simulink model "model_am_scalar"  (R2025a)
settings: Solver=FixedStepAuto  StartTime=0.0  StopTime=6  FixedStep=0.0001  RelTol=1e-3
values from neighbouring files (symbols this model uses):
  f = 50    [parametres_AM.m]
  J = 0.00096 * 5    (= 0.0048)    [parametres_AM.m]
  L1 = Lh + L1sig    (= 0.579)    [parametres_AM.m]
  L2 = L1    (= 0.579)    [parametres_AM.m]
  Lh = 0.56    [parametres_AM.m]
  M = 3.7    [parametres_AM.m]
  p = 2    [parametres_AM.m]
  R1 = 7.03    [parametres_AM.m]
  R2 = 3.44    [parametres_AM.m]
  sig = 1 - (Lh^2 / (L1 * L2))    (= 0.0645535599763)    [parametres_AM.m]
  U = 380    [parametres_AM.m]
  w = 2 * pi / 60 * n    (= 297.40410454)    [parametres_AM.m]
libraries: simulink x1
settings Model: Creator=Kajo  LastModifiedBy=emaka
settings SolverCC: AlgebraicLoopSolver=TrustRegion
settings DataIOCC: SaveOutput=off  SignalLogging=off  DSMLogging=off  SaveTime=off  ReturnWorkspaceOutputs=off
settings DebuggingCC: UnconnectedInputMsg=warning  UnconnectedOutputMsg=warning  UnconnectedLineMsg=warning
settings ModelReferenceCC: EnableRefExpFcnMdlSchedulingChecks=on
settings RTWCC: GPUComputeCapability=3.5

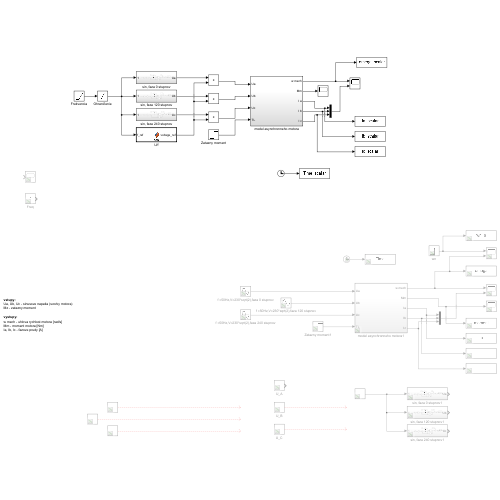
[thumbnail: Simulink's stored preview of the top-level diagram]
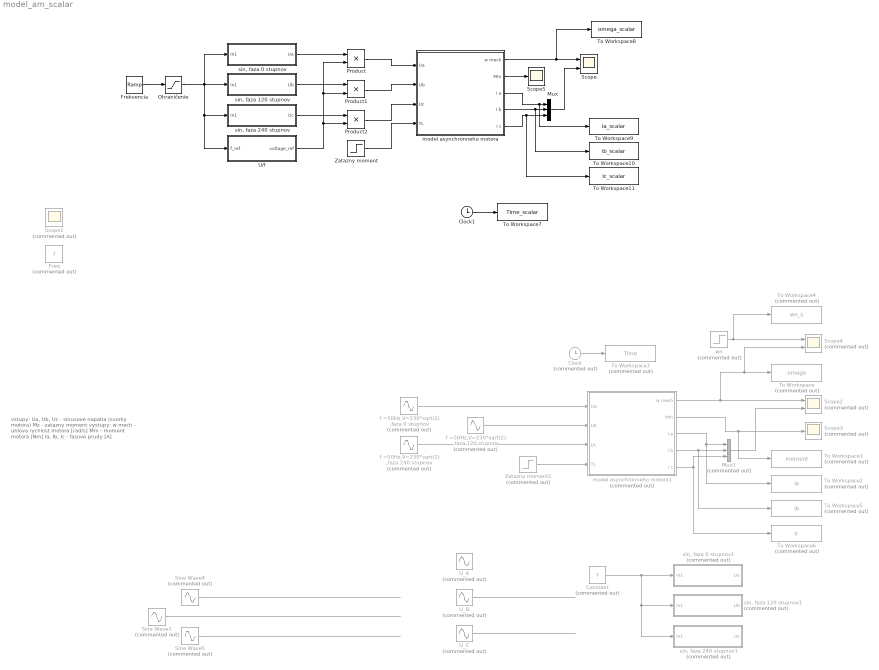
== system model_am_scalar ==
  note: vstupy:
      | Ua, Ub, Uc - sinusove napatia (svorky motora)
      | Mz - zatazny moment
      |
      | vystupy:
      | w mech - uhlova rychlost motora [rad/s]
      | Mm - moment motora [Nm]
      | Ia, Ib, Ic - fazove prudy [A]
  Clock : Clock  Commented=on
  Clock1 : Clock
  Constant : Constant  Commented=on  Value=f
  Frekvencia : simulink/Sources/Ramp  slope=16.67  start=0  InitialOutput=0
  Freq : Constant  Commented=on  Value=f  SampleTime=-1
  Mux : Mux  Inputs=3
  Mux1 : Mux  Commented=on  Inputs=3
  Ohraničenie : Saturate  UpperLimit=50  LowerLimit=0
  Product : Product
  Product1 : Product
  Product2 : Product
  Scope : Scope  NumInputPorts=2
      settings: ActiveDisplayYMinimum=-39.249692193358051  ActiveDisplayYMaximum=353.24722973603127
  Scope1 : Scope  Commented=on
      settings: ActiveDisplayYMinimum=-474.99354  ActiveDisplayYMaximum=474.99354
  Scope2 : Scope  Commented=on  NumInputPorts=2
      settings: ActiveDisplayYMinimum=-42.752099667675139  ActiveDisplayYMaximum=384.76889700905195  DataLoggingVariableName=ScopeData2
  Scope3 : Scope  Commented=on
      settings: ActiveDisplayYMinimum=-5.36519948546464  ActiveDisplayYMaximum=9.1078949851070767  DataLoggingVariableName=ScopeData3
  Scope4 : Scope  Commented=on  NumInputPorts=2
      settings: ActiveDisplayYMinimum=-1  ActiveDisplayYMaximum=1  DataLoggingVariableName=ScopeData4
  Scope5 : Scope
      settings: ActiveDisplayYMinimum=-0.94302291476539146  ActiveDisplayYMaximum=6.8461974059392778  DataLoggingVariableName=ScopeData6
  Sine Wave3 : Sin  Commented=on  Amplitude=U  Frequency=2*pi*50  SampleTime=0
  Sine Wave4 : Sin  Commented=on  Amplitude=U  Frequency=2*pi*50  Phase=(2*pi)/3  SampleTime=0
  Sine Wave5 : Sin  Commented=on  Amplitude=U  Frequency=2*pi*50  Phase=-(2*pi)/3  SampleTime=0
  To Workspace : ToWorkspace  Commented=on  VariableName=omega  SampleTime=-1
  To Workspace1 : ToWorkspace  Commented=on  VariableName=moment  SampleTime=-1
  To Workspace10 : ToWorkspace  VariableName=ib_scalar  SampleTime=-1
  To Workspace11 : ToWorkspace  VariableName=ic_scalar  SampleTime=-1
  To Workspace2 : ToWorkspace  Commented=on  VariableName=ia  SampleTime=-1
  To Workspace3 : ToWorkspace  Commented=on  VariableName=Time  SampleTime=-1
      settings: Save2DSignal=2-D array (concatenate along first dimension)
  To Workspace4 : ToWorkspace  Commented=on  VariableName=wn_s  SampleTime=-1
      settings: Save2DSignal=2-D array (concatenate along first dimension)
  To Workspace5 : ToWorkspace  Commented=on  VariableName=ib  SampleTime=-1
  To Workspace6 : ToWorkspace  Commented=on  VariableName=ic  SampleTime=-1
  To Workspace7 : ToWorkspace  VariableName=Time_scalar  SampleTime=-1
      settings: Save2DSignal=2-D array (concatenate along first dimension)
  To Workspace8 : ToWorkspace  VariableName=omega_scalar  SampleTime=-1
  To Workspace9 : ToWorkspace  VariableName=ia_scalar  SampleTime=-1
  U/f : MATLAB Function  TreatAsAtomicUnit=on
  U_A : Sin  Commented=on  Amplitude=U  Frequency=2*pi*f  SampleTime=0
  U_B : Sin  Commented=on  Amplitude=U  Frequency=2*pi*f  Phase=(2*pi)/3  SampleTime=0
  U_C : Sin  Commented=on  Amplitude=U  Frequency=2*pi*f  Phase=-(2*pi)/3  SampleTime=0
  Zatazny moment : Step  Time=4  After=M  SampleTime=0
  Zatazny moment1 : Step  Commented=on  After=M  SampleTime=0
  f =50Hz,V=230*sqrt(2),faza 0 stupnov : Sin  Commented=on  Amplitude=230*sqrt(2)  Frequency=2*pi*f  SampleTime=0
  f =50Hz,V=230*sqrt(2),faza 120 stupnov : Sin  Commented=on  Amplitude=230*sqrt(2)  Frequency=2*pi*f  Phase=-2*pi/3  SampleTime=0
  f =50Hz,V=230*sqrt(2),faza 240 stupnov : Sin  Commented=on  Amplitude=230*sqrt(2)  Frequency=2*pi*f  Phase=-4*pi/3  SampleTime=0
  model asynchronneho motora : Subsystem
  model asynchronneho motora1 : Subsystem  Commented=on
  "sin, faza 0 stupnov" : Subsystem
  "sin, faza 0 stupnov1" : Subsystem  Commented=on
  "sin, faza 120 stupnov" : Subsystem
  "sin, faza 120 stupnov1" : Subsystem  Commented=on
  "sin, faza 240 stupnov" : Subsystem
  "sin, faza 240 stupnov1" : Subsystem  Commented=on
  wn : Step  Commented=on  Time=0.01  After=w  SampleTime=0
  wires:
  Zatazny moment/1 -> model asynchronneho motora/4(TL)
  model asynchronneho motora/3(I a) -> To Workspace9/1, Mux/1
  model asynchronneho motora/4(I b) -> To Workspace10/1, Mux/2
  model asynchronneho motora/5(I c) -> To Workspace11/1, Mux/3
  Mux/1 -> Scope/2
  Product/1 -> model asynchronneho motora/1(Ua)
  Product1/1 -> model asynchronneho motora/2(Ub)
  Product2/1 -> model asynchronneho motora/3(Uc)
  "sin, faza 0 stupnov"/1(Ua) -> Product/1
  "sin, faza 120 stupnov"/1(Ub) -> Product1/1
  "sin, faza 240 stupnov"/1(Uc) -> Product2/1
  Ohraničenie/1 -> "sin, faza 0 stupnov"/1(In1), U/f/1(f_ref), "sin, faza 240 stupnov"/1(In1), "sin, faza 120 stupnov"/1(In1)
  Frekvencia/1 -> Ohraničenie/1
  U/f/1(voltage_ref) -> Product/2, Product1/2, Product2/2
  model asynchronneho motora1/4(I b) -> To Workspace5/1, Mux1/2
  model asynchronneho motora1/3(I a) -> Mux1/1, To Workspace2/1
  model asynchronneho motora1/5(I c) -> To Workspace6/1, Mux1/3
  Zatazny moment1/1 -> model asynchronneho motora1/4(TL)
  model asynchronneho motora1/1(w mech) -> Scope4/2, To Workspace/1, Scope2/1
  Mux1/1 -> Scope2/2
  U_C/1 -> ?
  U_B/1 -> ?
  Constant/1 -> "sin, faza 240 stupnov1"/1(In1), "sin, faza 120 stupnov1"/1(In1), "sin, faza 0 stupnov1"/1(In1)
  model asynchronneho motora1/2(Mm) -> To Workspace1/1, Scope3/1
  Sine Wave4/1 -> ?
  Sine Wave5/1 -> ?
  Sine Wave3/1 -> ?
  f =50Hz,V=230*sqrt(2),faza 0 stupnov/1 -> model asynchronneho motora1/1(Ua)
  f =50Hz,V=230*sqrt(2),faza 120 stupnov/1 -> model asynchronneho motora1/2(Ub)
  f =50Hz,V=230*sqrt(2),faza 240 stupnov/1 -> model asynchronneho motora1/3(Uc)
  wn/1 -> To Workspace4/1, Scope4/1
  Clock/1 -> To Workspace3/1
  model asynchronneho motora/2(Mm) -> Scope5/1
  Clock1/1 -> To Workspace7/1
  model asynchronneho motora/1(w mech) -> To Workspace8/1, Scope/1

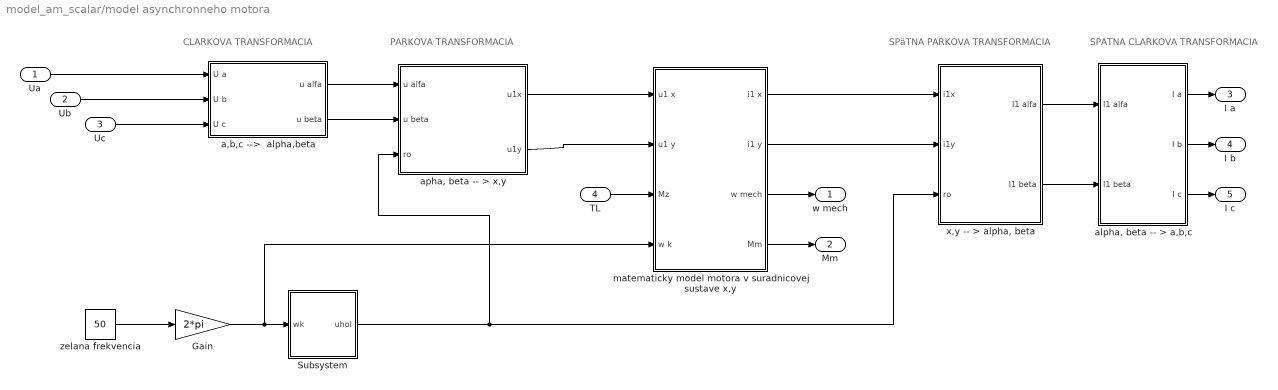
== system model_am_scalar/model asynchronneho motora ==
  note: PARKOVA TRANSFORMACIA
  note: SPATNA CLARKOVA TRANSFORMACIA
  note: SPäTNA PARKOVA TRANSFORMACIA
  note: CLARKOVA TRANSFORMACIA
  Ua : Inport
  Ub : Inport  Port=2
  Uc : Inport  Port=3
  TL : Inport  Port=4
  Gain : Gain  Gain=2*pi
  Subsystem : Subsystem
  "a,b,c -->  alpha,beta " : Subsystem
  "alpha, beta -- > a,b,c" : Subsystem
  "apha, beta -- > x,y" : Subsystem
  matematicky model motora v suradnicovej sustave x,y : Subsystem
  "x,y -- > alpha, beta" : Subsystem
  zelana frekvencia : Constant  Value=50
  w mech : Outport
  Mm : Outport  Port=2
  I a : Outport  Port=3
  I b : Outport  Port=4
  I c : Outport  Port=5
  wires:
  "a,b,c -->  alpha,beta "/1(u alfa) -> "apha, beta -- > x,y"/1(u alfa)
  "a,b,c -->  alpha,beta "/2(u beta) -> "apha, beta -- > x,y"/2(u beta)
  "apha, beta -- > x,y"/1(u1x) -> matematicky model motora v suradnicovej sustave x,y/1(u1 x)
  "apha, beta -- > x,y"/2(u1y) -> matematicky model motora v suradnicovej sustave x,y/2(u1 y)
  "x,y -- > alpha, beta"/1(I1 alfa) -> "alpha, beta -- > a,b,c"/1(I1 alfa)
  "x,y -- > alpha, beta"/2(I1 beta) -> "alpha, beta -- > a,b,c"/2(I1 beta)
  "alpha, beta -- > a,b,c"/1(I a) -> I a/1
  "alpha, beta -- > a,b,c"/2(I b) -> I b/1
  "alpha, beta -- > a,b,c"/3(I c) -> I c/1
  Ua/1 -> "a,b,c -->  alpha,beta "/1(U a)
  Ub/1 -> "a,b,c -->  alpha,beta "/2(U b)
  Uc/1 -> "a,b,c -->  alpha,beta "/3(U c)
  TL/1 -> matematicky model motora v suradnicovej sustave x,y/3(Mz)
  matematicky model motora v suradnicovej sustave x,y/2(i1 y) -> "x,y -- > alpha, beta"/2(i1y)
  matematicky model motora v suradnicovej sustave x,y/3(w mech) -> w mech/1
  matematicky model motora v suradnicovej sustave x,y/4(Mm) -> Mm/1
  matematicky model motora v suradnicovej sustave x,y/1(i1 x) -> "x,y -- > alpha, beta"/1(i1x)
  zelana frekvencia/1 -> Gain/1
  Gain/1 -> matematicky model motora v suradnicovej sustave x,y/4(w k), Subsystem/1(wk)
  Subsystem/1(uhol) -> "apha, beta -- > x,y"/3(ro), "x,y -- > alpha, beta"/3("ro ")

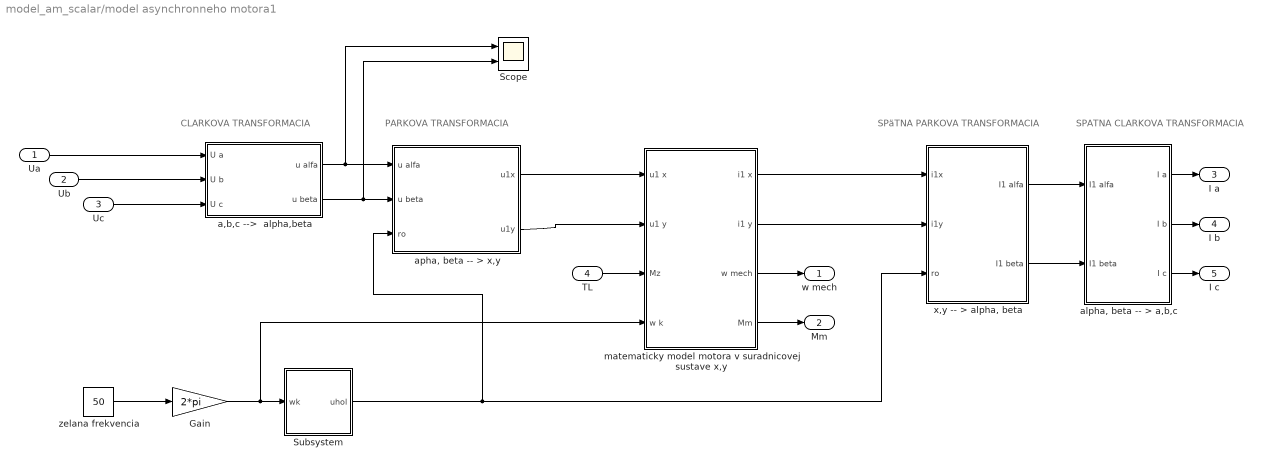
== system model_am_scalar/model asynchronneho motora1 ==
  note: PARKOVA TRANSFORMACIA
  note: SPATNA CLARKOVA TRANSFORMACIA
  note: SPäTNA PARKOVA TRANSFORMACIA
  note: CLARKOVA TRANSFORMACIA
  Ua : Inport
  Ub : Inport  Port=2
  Uc : Inport  Port=3
  TL : Inport  Port=4
  Gain : Gain  Gain=2*pi
  Scope : Scope  NumInputPorts=2
      settings: ActiveDisplayYMinimum=-412.2715694519627  ActiveDisplayYMaximum=371.70919052872546  DataLoggingVariableName=ScopeData5
  Subsystem : Subsystem
  "a,b,c -->  alpha,beta " : Subsystem
  "alpha, beta -- > a,b,c" : Subsystem
  "apha, beta -- > x,y" : Subsystem
  matematicky model motora v suradnicovej sustave x,y : Subsystem
  "x,y -- > alpha, beta" : Subsystem
  zelana frekvencia : Constant  Value=50
  w mech : Outport
  Mm : Outport  Port=2
  I a : Outport  Port=3
  I b : Outport  Port=4
  I c : Outport  Port=5
  wires:
  "a,b,c -->  alpha,beta "/1(u alfa) -> Scope/1, "apha, beta -- > x,y"/1(u alfa)
  "a,b,c -->  alpha,beta "/2(u beta) -> Scope/2, "apha, beta -- > x,y"/2(u beta)
  "apha, beta -- > x,y"/1(u1x) -> matematicky model motora v suradnicovej sustave x,y/1(u1 x)
  "apha, beta -- > x,y"/2(u1y) -> matematicky model motora v suradnicovej sustave x,y/2(u1 y)
  "x,y -- > alpha, beta"/1(I1 alfa) -> "alpha, beta -- > a,b,c"/1(I1 alfa)
  "x,y -- > alpha, beta"/2(I1 beta) -> "alpha, beta -- > a,b,c"/2(I1 beta)
  "alpha, beta -- > a,b,c"/1(I a) -> I a/1
  "alpha, beta -- > a,b,c"/2(I b) -> I b/1
  "alpha, beta -- > a,b,c"/3(I c) -> I c/1
  Ua/1 -> "a,b,c -->  alpha,beta "/1(U a)
  Ub/1 -> "a,b,c -->  alpha,beta "/2(U b)
  Uc/1 -> "a,b,c -->  alpha,beta "/3(U c)
  TL/1 -> matematicky model motora v suradnicovej sustave x,y/3(Mz)
  matematicky model motora v suradnicovej sustave x,y/2(i1 y) -> "x,y -- > alpha, beta"/2(i1y)
  matematicky model motora v suradnicovej sustave x,y/3(w mech) -> w mech/1
  matematicky model motora v suradnicovej sustave x,y/4(Mm) -> Mm/1
  matematicky model motora v suradnicovej sustave x,y/1(i1 x) -> "x,y -- > alpha, beta"/1(i1x)
  zelana frekvencia/1 -> Gain/1
  Gain/1 -> matematicky model motora v suradnicovej sustave x,y/4(w k), Subsystem/1(wk)
  Subsystem/1(uhol) -> "apha, beta -- > x,y"/3(ro), "x,y -- > alpha, beta"/3("ro ")

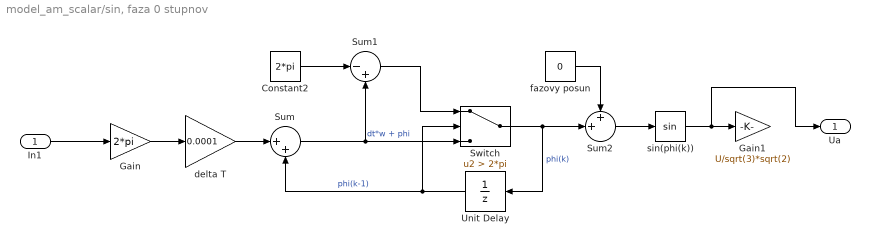
== system model_am_scalar/sin, faza 0 stupnov ==
  In1 : Inport
  Constant2 : Constant  Value=2*pi  SampleTime=-1
  Gain : Gain  Gain=2*pi
  Gain1 : Gain  Gain=U/sqrt(3)*sqrt(2)
  Sum : Sum  Inputs=|++
  Sum1 : Sum  Inputs=|-+
  Sum2 : Sum  Inputs=++|
  Switch : Switch  Criteria=u2 > Threshold  Threshold=2*pi  SaturateOnIntegerOverflow=off  InputSameDT=off
  Unit Delay : UnitDelay  SampleTime=-1  HasFrameUpgradeWarning=on
  delta T : Gain  Gain=0.0001
  fazovy posun : Constant  Value=0  SampleTime=-1
  sin(phi(k)) : Trigonometry
  Ua : Outport
  wires:
  Sum2/1 -> sin(phi(k))/1
  Switch/1 -> Sum2/2, Unit Delay/1  "phi(k)"
  delta T/1 -> Sum/1
  Sum/1 -> Switch/3, Sum1/2  "dt*w + phi"
  Gain/1 -> delta T/1
  Constant2/1 -> Sum1/1
  Unit Delay/1 -> Sum/2, Switch/2  "phi(k-1)"
  Sum1/1 -> Switch/1
  fazovy posun/1 -> Sum2/1
  In1/1 -> Gain/1
  sin(phi(k))/1 -> Ua/1, Gain1/1

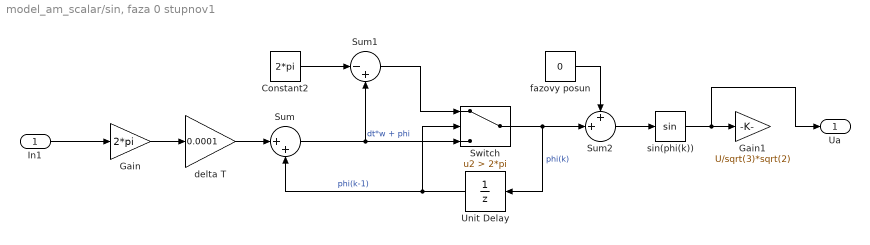
== system model_am_scalar/sin, faza 0 stupnov1 ==
  In1 : Inport
  Constant2 : Constant  Value=2*pi  SampleTime=-1
  Gain : Gain  Gain=2*pi
  Gain1 : Gain  Gain=U/sqrt(3)*sqrt(2)
  Sum : Sum  Inputs=|++
  Sum1 : Sum  Inputs=|-+
  Sum2 : Sum  Inputs=++|
  Switch : Switch  Criteria=u2 > Threshold  Threshold=2*pi  SaturateOnIntegerOverflow=off  InputSameDT=off
  Unit Delay : UnitDelay  SampleTime=-1  HasFrameUpgradeWarning=on
  delta T : Gain  Gain=0.0001
  fazovy posun : Constant  Value=0  SampleTime=-1
  sin(phi(k)) : Trigonometry
  Ua : Outport
  wires:
  Sum2/1 -> sin(phi(k))/1
  Switch/1 -> Sum2/2, Unit Delay/1  "phi(k)"
  delta T/1 -> Sum/1
  Sum/1 -> Switch/3, Sum1/2  "dt*w + phi"
  Gain/1 -> delta T/1
  Constant2/1 -> Sum1/1
  Unit Delay/1 -> Sum/2, Switch/2  "phi(k-1)"
  Sum1/1 -> Switch/1
  fazovy posun/1 -> Sum2/1
  In1/1 -> Gain/1
  sin(phi(k))/1 -> Ua/1, Gain1/1

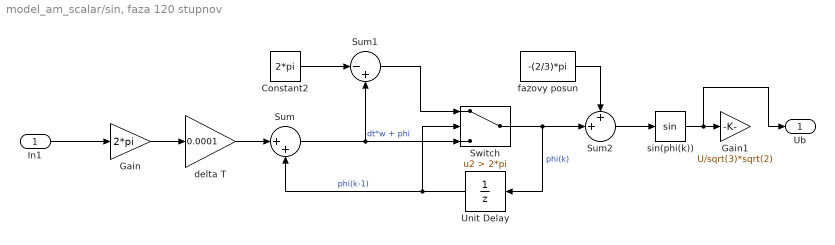
== system model_am_scalar/sin, faza 120 stupnov ==
  In1 : Inport
  Constant2 : Constant  Value=2*pi  SampleTime=-1
  Gain : Gain  Gain=2*pi
  Gain1 : Gain  Gain=U/sqrt(3)*sqrt(2)
  Sum : Sum  Inputs=|++
  Sum1 : Sum  Inputs=|-+
  Sum2 : Sum  Inputs=++|
  Switch : Switch  Criteria=u2 > Threshold  Threshold=2*pi  SaturateOnIntegerOverflow=off  InputSameDT=off
  Unit Delay : UnitDelay  SampleTime=-1  HasFrameUpgradeWarning=on
  delta T : Gain  Gain=0.0001
  fazovy posun : Constant  Value=-(2/3)*pi  SampleTime=-1
  sin(phi(k)) : Trigonometry
  Ub : Outport
  wires:
  Sum2/1 -> sin(phi(k))/1
  Switch/1 -> Sum2/2, Unit Delay/1  "phi(k)"
  delta T/1 -> Sum/1
  Sum/1 -> Switch/3, Sum1/2  "dt*w + phi"
  Gain/1 -> delta T/1
  Constant2/1 -> Sum1/1
  Unit Delay/1 -> Sum/2, Switch/2  "phi(k-1)"
  Sum1/1 -> Switch/1
  fazovy posun/1 -> Sum2/1
  In1/1 -> Gain/1
  sin(phi(k))/1 -> Ub/1, Gain1/1

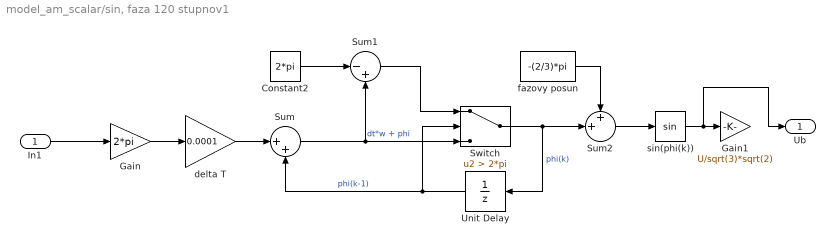
== system model_am_scalar/sin, faza 120 stupnov1 ==
  In1 : Inport
  Constant2 : Constant  Value=2*pi  SampleTime=-1
  Gain : Gain  Gain=2*pi
  Gain1 : Gain  Gain=U/sqrt(3)*sqrt(2)
  Sum : Sum  Inputs=|++
  Sum1 : Sum  Inputs=|-+
  Sum2 : Sum  Inputs=++|
  Switch : Switch  Criteria=u2 > Threshold  Threshold=2*pi  SaturateOnIntegerOverflow=off  InputSameDT=off
  Unit Delay : UnitDelay  SampleTime=-1  HasFrameUpgradeWarning=on
  delta T : Gain  Gain=0.0001
  fazovy posun : Constant  Value=-(2/3)*pi  SampleTime=-1
  sin(phi(k)) : Trigonometry
  Ub : Outport
  wires:
  Sum2/1 -> sin(phi(k))/1
  Switch/1 -> Sum2/2, Unit Delay/1  "phi(k)"
  delta T/1 -> Sum/1
  Sum/1 -> Switch/3, Sum1/2  "dt*w + phi"
  Gain/1 -> delta T/1
  Constant2/1 -> Sum1/1
  Unit Delay/1 -> Sum/2, Switch/2  "phi(k-1)"
  Sum1/1 -> Switch/1
  fazovy posun/1 -> Sum2/1
  In1/1 -> Gain/1
  sin(phi(k))/1 -> Ub/1, Gain1/1

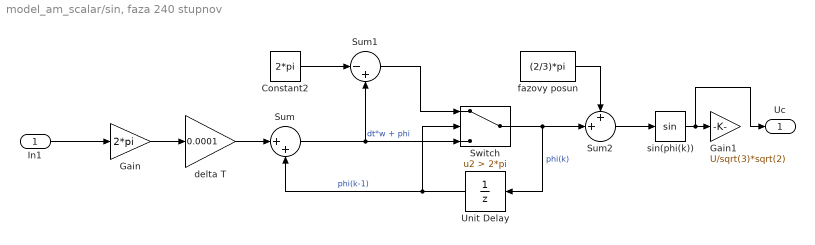
== system model_am_scalar/sin, faza 240 stupnov ==
  In1 : Inport
  Constant2 : Constant  Value=2*pi  SampleTime=-1
  Gain : Gain  Gain=2*pi
  Gain1 : Gain  Gain=U/sqrt(3)*sqrt(2)
  Sum : Sum  Inputs=|++
  Sum1 : Sum  Inputs=|-+
  Sum2 : Sum  Inputs=++|
  Switch : Switch  Criteria=u2 > Threshold  Threshold=2*pi  SaturateOnIntegerOverflow=off  InputSameDT=off
  Unit Delay : UnitDelay  SampleTime=-1  HasFrameUpgradeWarning=on
  delta T : Gain  Gain=0.0001
  fazovy posun : Constant  Value=(2/3)*pi  SampleTime=-1
  sin(phi(k)) : Trigonometry
  Uc : Outport
  wires:
  Sum2/1 -> sin(phi(k))/1
  Switch/1 -> Sum2/2, Unit Delay/1  "phi(k)"
  delta T/1 -> Sum/1
  Sum/1 -> Switch/3, Sum1/2  "dt*w + phi"
  Gain/1 -> delta T/1
  Constant2/1 -> Sum1/1
  Unit Delay/1 -> Sum/2, Switch/2  "phi(k-1)"
  Sum1/1 -> Switch/1
  fazovy posun/1 -> Sum2/1
  In1/1 -> Gain/1
  sin(phi(k))/1 -> Uc/1, Gain1/1

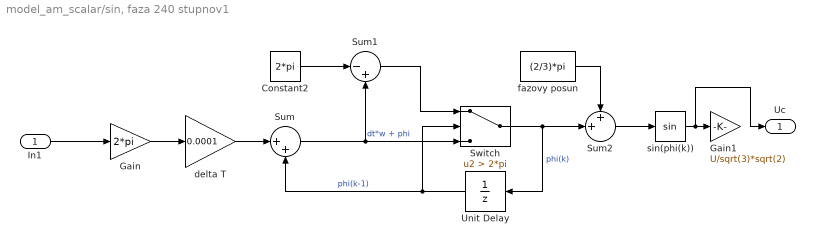
== system model_am_scalar/sin, faza 240 stupnov1 ==
  In1 : Inport
  Constant2 : Constant  Value=2*pi  SampleTime=-1
  Gain : Gain  Gain=2*pi
  Gain1 : Gain  Gain=U/sqrt(3)*sqrt(2)
  Sum : Sum  Inputs=|++
  Sum1 : Sum  Inputs=|-+
  Sum2 : Sum  Inputs=++|
  Switch : Switch  Criteria=u2 > Threshold  Threshold=2*pi  SaturateOnIntegerOverflow=off  InputSameDT=off
  Unit Delay : UnitDelay  SampleTime=-1  HasFrameUpgradeWarning=on
  delta T : Gain  Gain=0.0001
  fazovy posun : Constant  Value=(2/3)*pi  SampleTime=-1
  sin(phi(k)) : Trigonometry
  Uc : Outport
  wires:
  Sum2/1 -> sin(phi(k))/1
  Switch/1 -> Sum2/2, Unit Delay/1  "phi(k)"
  delta T/1 -> Sum/1
  Sum/1 -> Switch/3, Sum1/2  "dt*w + phi"
  Gain/1 -> delta T/1
  Constant2/1 -> Sum1/1
  Unit Delay/1 -> Sum/2, Switch/2  "phi(k-1)"
  Sum1/1 -> Switch/1
  fazovy posun/1 -> Sum2/1
  In1/1 -> Gain/1
  sin(phi(k))/1 -> Uc/1, Gain1/1

== system model_am_scalar/model asynchronneho motora/Subsystem ==
  note: phi (k-1)
  note: dt*w + phi
  note: w(k)
  note: phi (k)
  wk : Inport
  Sum1 : Sum  Inputs=-+
  Sum2 : Sum
  Switch : Switch  Criteria=u2 > Threshold  Threshold=2*pi  OutDataTypeStr=single  SaturateOnIntegerOverflow=off  InputSameDT=off
  Unit Delay1 : UnitDelay  SampleTime=-1  HasFrameUpgradeWarning=on
  delta T : Gain  Gain=0.0001  OutDataTypeStr=Inherit: Same as input
  faza2 : Constant  Value=2*pi  OutDataTypeStr=single
  uhol : Outport
  wires:
  Switch/1 -> uhol/1, Unit Delay1/1
  delta T/1 -> Sum2/1
  Sum2/1 -> Switch/3, Sum1/2
  Unit Delay1/1 -> Switch/2, Sum2/2
  Sum1/1 -> Switch/1
  wk/1 -> delta T/1
  faza2/1 -> Sum1/1

== system model_am_scalar/model asynchronneho motora/a,b,c -->  alpha,beta  ==
  U a : Inport
  U b : Inport  Port=2
  U c : Inport  Port=3
  1/sqrt(3) : Gain  Gain=1/sqrt(3)
  Sum : Sum  Inputs=|+-
  u alfa : Outport
  u beta : Outport  Port=2
  wires:
  U b/1 -> Sum/1
  U c/1 -> Sum/2
  1/sqrt(3)/1 -> u beta/1
  U a/1 -> u alfa/1
  Sum/1 -> 1/sqrt(3)/1

== system model_am_scalar/model asynchronneho motora/alpha, beta -- > a,b,c ==
  note: sqrt(3)/2
  I1 alfa : Inport
  I1 beta : Inport  Port=2
  Gain : Gain  Gain=0.5
  Gain1 : Gain  Gain=sqrt(3)/2
  Sum : Sum  Inputs=-+
  Sum1 : Sum  Inputs=--
  I a : Outport
  I b : Outport  Port=2
  I c : Outport  Port=3
  wires:
  Sum1/1 -> I c/1
  Gain1/1 -> Sum1/2, Sum/2
  I1 beta/1 -> Gain1/1
  Sum/1 -> I b/1
  Gain/1 -> Sum1/1, Sum/1
  I1 alfa/1 -> I a/1, Gain/1

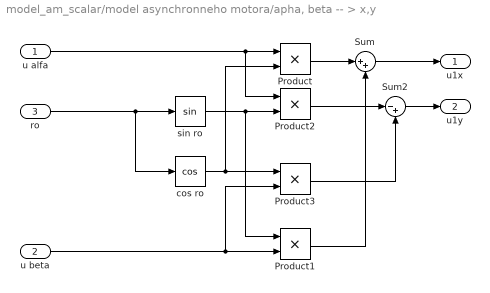
== system model_am_scalar/model asynchronneho motora/apha, beta -- > x,y ==
  u alfa : Inport
  u beta : Inport  Port=2
  ro : Inport  Port=3
  Product{,1..3} (4 alike) : Product  RndMeth=Zero
  Sum : Sum  Inputs=|++
  Sum2 : Sum  Inputs=|-+
  cos ro : Trigonometry  Operator=cos
  sin ro : Trigonometry
  u1x : Outport
  u1y : Outport  Port=2
  wires:
  Product3/1 -> Sum2/2
  Sum2/1 -> u1y/1
  Product2/1 -> Sum2/1
  Sum/1 -> u1x/1
  Product1/1 -> Sum/2
  Product/1 -> Sum/1
  u beta/1 -> Product1/2, Product3/2
  sin ro/1 -> Product2/2, Product1/1
  u alfa/1 -> Product/1, Product2/1
  cos ro/1 -> Product3/1, Product/2
  ro/1 -> sin ro/1, cos ro/1

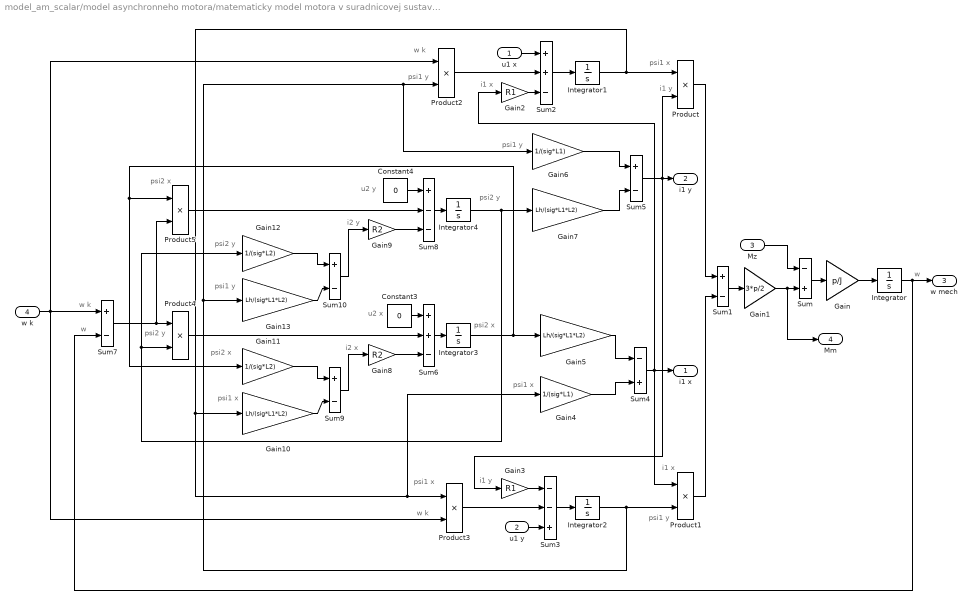
== system model_am_scalar/model asynchronneho motora/matematicky model motora v suradnicovej sustave x,y ==
  note: w
  note: psi1 x
  note: i1 y
  note: psi1 y
  note: i1 x
  note: i1 x
  note: w k
  note: psi1 y
  note: i1 y
  note: w k
  note: psi1 x
  note: psi1 x
  note: psi2 x
  note: psi1 y
  note: psi2 y
  note: u2 x
  note: i2 x
  note: psi2 y
  note: w
  note: i2 y
  note: u2 y
  note: psi2 x
  note: psi1 x
  note: psi2 x
  note: psi2 y
  note: psi1 y
  note: w k
  u1 x : Inport
  u1 y : Inport  Port=2
  Mz : Inport  Port=3
  w k : Inport  Port=4
  Constant3 : Constant  Value=0
  Constant4 : Constant  Value=0
  Gain : Gain  Gain=p/J
  Gain1 : Gain  Gain=3*p/2
  Gain{5,7,10,13} (4 alike) : Gain  Gain=Lh/(sig*L1*L2)
  Gain11 : Gain  Gain=1/(sig*L2)
  Gain12 : Gain  Gain=1/(sig*L2)
  Gain2 : Gain  Gain=R1
  Gain3 : Gain  Gain=R1
  Gain4 : Gain  Gain=1/(sig*L1)
  Gain6 : Gain  Gain=1/(sig*L1)
  Gain8 : Gain  Gain=R2
  Gain9 : Gain  Gain=R2
  Integrator{,1..4} (5 alike) : Integrator
  Product{,1..5} (6 alike) : Product  RndMeth=Zero
  Sum : Sum  Inputs=-+
  Sum{1,5,7,9..10} (5 alike) : Sum  Inputs=+-
  Sum2 : Sum  Inputs=++-
  Sum3 : Sum  Inputs=--+
  Sum4 : Sum  Inputs=-+
  Sum6 : Sum  Inputs=++-
  Sum8 : Sum  Inputs=+--
  i1 x : Outport
  i1 y : Outport  Port=2
  w mech : Outport  Port=3
  Mm : Outport  Port=4
  wires:
  Gain/1 -> Integrator/1
  Sum/1 -> Gain/1
  Sum1/1 -> Gain1/1
  Gain1/1 -> Sum/2, Mm/1
  Integrator/1 -> Sum7/2, w mech/1
  Product/1 -> Sum1/1
  Product1/1 -> Sum1/2
  Integrator1/1 -> Product/1, Gain10/1, Product3/1, Gain4/1
  Integrator2/1 -> Product1/2, Gain13/1, Product2/2, Gain6/1
  Sum2/1 -> Integrator1/1
  Sum3/1 -> Integrator2/1
  Gain2/1 -> Sum2/3
  Product2/1 -> Sum2/2
  u1 x/1 -> Sum2/1
  Product3/1 -> Sum3/2
  Sum4/1 -> Gain2/1, i1 x/1, Product1/1
  Gain5/1 -> Sum4/1
  Gain6/1 -> Sum5/1
  Sum5/1 -> Product/2, Gain3/1, i1 y/1
  Gain7/1 -> Sum5/2
  Integrator3/1 -> Gain5/1, Product5/1, Gain11/1
  Integrator4/1 -> Gain7/1, Product4/2, Gain12/1
  Sum6/1 -> Integrator3/1
  Constant3/1 -> Sum6/1
  Gain8/1 -> Sum6/3
  Product4/1 -> Sum6/2
  Sum7/1 -> Product5/2, Product4/1
  Sum8/1 -> Integrator4/1
  Gain9/1 -> Sum8/3
  Constant4/1 -> Sum8/1
  Product5/1 -> Sum8/2
  Sum9/1 -> Gain8/1
  Gain10/1 -> Sum9/2
  Gain11/1 -> Sum9/1
  Sum10/1 -> Gain9/1
  Gain12/1 -> Sum10/1
  Gain13/1 -> Sum10/2
  w k/1 -> Product3/2, Product2/1, Sum7/1
  Gain4/1 -> Sum4/2
  u1 y/1 -> Sum3/3
  Gain3/1 -> Sum3/1
  Mz/1 -> Sum/1

== system model_am_scalar/model asynchronneho motora/x,y -- > alpha, beta ==
  i1x : Inport
  i1y : Inport  Port=2
  "ro " : Inport  Port=3
  Product{,1..3} (4 alike) : Product  RndMeth=Zero
  Sum : Sum  Inputs=|+-
  Sum2 : Sum  Inputs=|++
  cos ro : Trigonometry  Operator=cos
  sin ro : Trigonometry
  I1 alfa : Outport
  I1 beta : Outport  Port=2
  wires:
  Product1/1 -> Sum2/2
  Product3/1 -> Sum2/1
  Product2/1 -> Sum/2
  Product/1 -> Sum/1
  i1y/1 -> Product2/2, Product1/2
  sin ro/1 -> Product3/2, Product2/1
  cos ro/1 -> Product1/1, Product/2
  i1x/1 -> Product/1, Product3/1
  Sum2/1 -> I1 beta/1
  Sum/1 -> I1 alfa/1
  "ro "/1 -> cos ro/1, sin ro/1

== system model_am_scalar/model asynchronneho motora1/Subsystem ==
  note: phi (k-1)
  note: dt*w + phi
  note: w(k)
  note: phi (k)
  wk : Inport
  Sum1 : Sum  Inputs=-+
  Sum2 : Sum
  Switch : Switch  Criteria=u2 > Threshold  Threshold=2*pi  OutDataTypeStr=single  SaturateOnIntegerOverflow=off  InputSameDT=off
  Unit Delay1 : UnitDelay  SampleTime=-1  HasFrameUpgradeWarning=on
  delta T : Gain  Gain=0.0001  OutDataTypeStr=Inherit: Same as input
  faza2 : Constant  Value=2*pi  OutDataTypeStr=single
  uhol : Outport
  wires:
  Switch/1 -> uhol/1, Unit Delay1/1
  delta T/1 -> Sum2/1
  Sum2/1 -> Switch/3, Sum1/2
  Unit Delay1/1 -> Switch/2, Sum2/2
  Sum1/1 -> Switch/1
  wk/1 -> delta T/1
  faza2/1 -> Sum1/1

== system model_am_scalar/model asynchronneho motora1/a,b,c -->  alpha,beta  ==
  U a : Inport
  U b : Inport  Port=2
  U c : Inport  Port=3
  1/sqrt(3) : Gain  Gain=1/sqrt(3)
  Sum : Sum  Inputs=|+-
  u alfa : Outport
  u beta : Outport  Port=2
  wires:
  U b/1 -> Sum/1
  U c/1 -> Sum/2
  1/sqrt(3)/1 -> u beta/1
  U a/1 -> u alfa/1
  Sum/1 -> 1/sqrt(3)/1

== system model_am_scalar/model asynchronneho motora1/alpha, beta -- > a,b,c ==
  note: sqrt(3)/2
  I1 alfa : Inport
  I1 beta : Inport  Port=2
  Gain : Gain  Gain=0.5
  Gain1 : Gain  Gain=sqrt(3)/2
  Sum : Sum  Inputs=-+
  Sum1 : Sum  Inputs=--
  I a : Outport
  I b : Outport  Port=2
  I c : Outport  Port=3
  wires:
  Sum1/1 -> I c/1
  Gain1/1 -> Sum1/2, Sum/2
  I1 beta/1 -> Gain1/1
  Sum/1 -> I b/1
  Gain/1 -> Sum1/1, Sum/1
  I1 alfa/1 -> I a/1, Gain/1

== system model_am_scalar/model asynchronneho motora1/apha, beta -- > x,y ==
  u alfa : Inport
  u beta : Inport  Port=2
  ro : Inport  Port=3
  Product{,1..3} (4 alike) : Product  RndMeth=Zero
  Sum : Sum  Inputs=|++
  Sum2 : Sum  Inputs=|-+
  cos ro : Trigonometry  Operator=cos
  sin ro : Trigonometry
  u1x : Outport
  u1y : Outport  Port=2
  wires:
  Product3/1 -> Sum2/2
  Sum2/1 -> u1y/1
  Product2/1 -> Sum2/1
  Sum/1 -> u1x/1
  Product1/1 -> Sum/2
  Product/1 -> Sum/1
  u beta/1 -> Product1/2, Product3/2
  sin ro/1 -> Product2/2, Product1/1
  u alfa/1 -> Product/1, Product2/1
  cos ro/1 -> Product3/1, Product/2
  ro/1 -> sin ro/1, cos ro/1

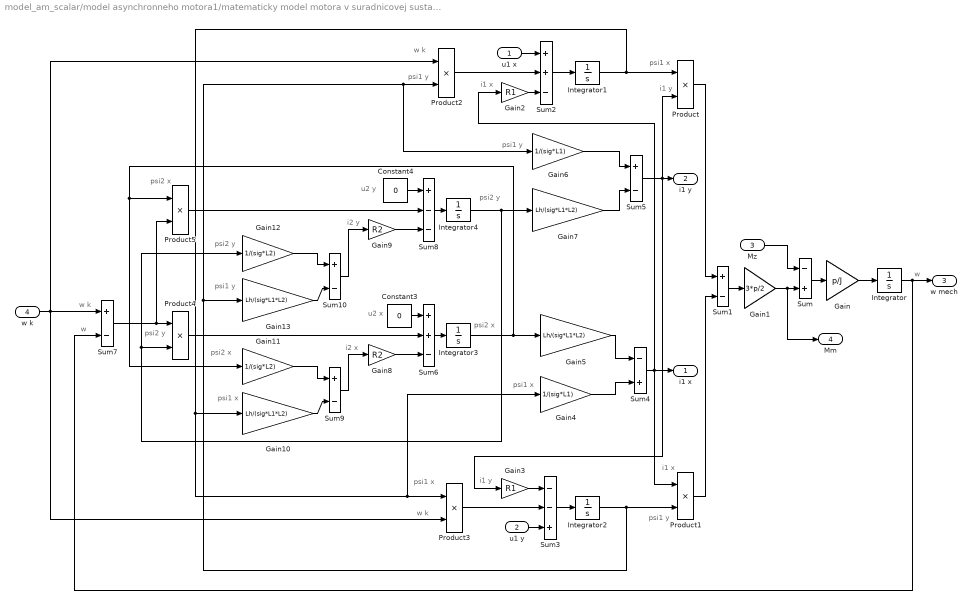
== system model_am_scalar/model asynchronneho motora1/matematicky model motora v suradnicovej sustave x,y ==
  note: w
  note: psi1 x
  note: i1 y
  note: psi1 y
  note: i1 x
  note: i1 x
  note: w k
  note: psi1 y
  note: i1 y
  note: w k
  note: psi1 x
  note: psi1 x
  note: psi2 x
  note: psi1 y
  note: psi2 y
  note: u2 x
  note: i2 x
  note: psi2 y
  note: w
  note: i2 y
  note: u2 y
  note: psi2 x
  note: psi1 x
  note: psi2 x
  note: psi2 y
  note: psi1 y
  note: w k
  u1 x : Inport
  u1 y : Inport  Port=2
  Mz : Inport  Port=3
  w k : Inport  Port=4
  Constant3 : Constant  Value=0
  Constant4 : Constant  Value=0
  Gain : Gain  Gain=p/J
  Gain1 : Gain  Gain=3*p/2
  Gain{5,7,10,13} (4 alike) : Gain  Gain=Lh/(sig*L1*L2)
  Gain11 : Gain  Gain=1/(sig*L2)
  Gain12 : Gain  Gain=1/(sig*L2)
  Gain2 : Gain  Gain=R1
  Gain3 : Gain  Gain=R1
  Gain4 : Gain  Gain=1/(sig*L1)
  Gain6 : Gain  Gain=1/(sig*L1)
  Gain8 : Gain  Gain=R2
  Gain9 : Gain  Gain=R2
  Integrator{,1..4} (5 alike) : Integrator
  Product{,1..5} (6 alike) : Product  RndMeth=Zero
  Sum : Sum  Inputs=-+
  Sum{1,5,7,9..10} (5 alike) : Sum  Inputs=+-
  Sum2 : Sum  Inputs=++-
  Sum3 : Sum  Inputs=--+
  Sum4 : Sum  Inputs=-+
  Sum6 : Sum  Inputs=++-
  Sum8 : Sum  Inputs=+--
  i1 x : Outport
  i1 y : Outport  Port=2
  w mech : Outport  Port=3
  Mm : Outport  Port=4
  wires:
  Gain/1 -> Integrator/1
  Sum/1 -> Gain/1
  Sum1/1 -> Gain1/1
  Gain1/1 -> Sum/2, Mm/1
  Integrator/1 -> Sum7/2, w mech/1
  Product/1 -> Sum1/1
  Product1/1 -> Sum1/2
  Integrator1/1 -> Product/1, Gain10/1, Product3/1, Gain4/1
  Integrator2/1 -> Product1/2, Gain13/1, Product2/2, Gain6/1
  Sum2/1 -> Integrator1/1
  Sum3/1 -> Integrator2/1
  Gain2/1 -> Sum2/3
  Product2/1 -> Sum2/2
  u1 x/1 -> Sum2/1
  Product3/1 -> Sum3/2
  Sum4/1 -> Gain2/1, i1 x/1, Product1/1
  Gain5/1 -> Sum4/1
  Gain6/1 -> Sum5/1
  Sum5/1 -> Product/2, Gain3/1, i1 y/1
  Gain7/1 -> Sum5/2
  Integrator3/1 -> Gain5/1, Product5/1, Gain11/1
  Integrator4/1 -> Gain7/1, Product4/2, Gain12/1
  Sum6/1 -> Integrator3/1
  Constant3/1 -> Sum6/1
  Gain8/1 -> Sum6/3
  Product4/1 -> Sum6/2
  Sum7/1 -> Product5/2, Product4/1
  Sum8/1 -> Integrator4/1
  Gain9/1 -> Sum8/3
  Constant4/1 -> Sum8/1
  Product5/1 -> Sum8/2
  Sum9/1 -> Gain8/1
  Gain10/1 -> Sum9/2
  Gain11/1 -> Sum9/1
  Sum10/1 -> Gain9/1
  Gain12/1 -> Sum10/1
  Gain13/1 -> Sum10/2
  w k/1 -> Product3/2, Product2/1, Sum7/1
  Gain4/1 -> Sum4/2
  u1 y/1 -> Sum3/3
  Gain3/1 -> Sum3/1
  Mz/1 -> Sum/1

== system model_am_scalar/model asynchronneho motora1/x,y -- > alpha, beta ==
  i1x : Inport
  i1y : Inport  Port=2
  "ro " : Inport  Port=3
  Product{,1..3} (4 alike) : Product  RndMeth=Zero
  Sum : Sum  Inputs=|+-
  Sum2 : Sum  Inputs=|++
  cos ro : Trigonometry  Operator=cos
  sin ro : Trigonometry
  I1 alfa : Outport
  I1 beta : Outport  Port=2
  wires:
  Product1/1 -> Sum2/2
  Product3/1 -> Sum2/1
  Product2/1 -> Sum/2
  Product/1 -> Sum/1
  i1y/1 -> Product2/2, Product1/2
  sin ro/1 -> Product3/2, Product2/1
  cos ro/1 -> Product1/1, Product/2
  i1x/1 -> Product/1, Product3/1
  Sum2/1 -> I1 beta/1
  Sum/1 -> I1 alfa/1
  "ro "/1 -> cos ro/1, sin ro/1

== matlab function model_am_scalar/U//f ==
  data: f_ref input; voltage_ref output
function voltage_ref = fcn(f_ref)
    % Параметры системы
    U_nom = 380;        % Номинальное напряжение (пример, можно изменить)
    f_nom = 50;         % Номинальная частота (50 Гц)
    U_boost = 20;       % Напряжение для низких частот
    f_boost = 3;        % Граница для Uboost

    % Логика зависимости амплитуды от частоты
    if f_ref <= f_boost
        voltage_ref = U_boost; % Для частот до 3 Гц - фиксированное напряжение U_boost
    elseif f_ref < f_nom
        voltage_ref = (U_nom / f_nom) * f_ref; % Линейное нарастание напряжения
    else
        voltage_ref = U_nom; % Для частот >= 50 Гц напряжение = U_nom
    end
end
